simulink model "levitador_mpc_ss_delta"  (Simulink 7.9)
settings: Solver=ode5  SolverMode=SingleTasking  StartTime=0.0  StopTime=2  FixedStep=0.001  RelTol=1e-3
values from neighbouring files (symbols this model uses):
  C = [1 0]    [parametros_maglev_ss.m]
  g = 9.8    [parametros_maglev_ss.m]
  gamma = 328    [parametros_maglev_ss.m]
  i0 = 0.514    [parametros_maglev_ss.m]
  Kdelta = aux2(1,:)    [matrizes_ss_delta.m]
  Kf = 1.2e-4    (= 0.00012)    [parametros_maglev_ss.m]
  mass = 2.12e-2    (= 0.0212)    [parametros_maglev_ss.m]
  Nu = aux(end,:)    [matrizes_ss_delta.m]
  Nx = aux(1:n,:)    [matrizes_ss_delta.m]
  r = 0.166    [parametros_maglev_ss.m]
  T = 0.005    [parametros_maglev_ss.m]
  up_equilibrio = ( sqrt(mass*g/Kf)*(yp_equilibrio - y0) / gamma - i0 ) / r    [parametros_maglev_ss.m]
  y0 = -7.47    [parametros_maglev_ss.m]
  yp_equilibrio = 0    [parametros_maglev_ss.m]
undefined symbols (not defined in the file or in its folder): A, B
settings Model: Creator=Kawakami  LastModifiedBy=Kawakami
settings DataIOCC: SignalLoggingName=sigsOut
settings OptimizationCC: BooleanDataType=off
settings DebuggingCC: SaveWithParameterizedLinksMsg=none  SignalResolutionControl=TryResolveAllWithWarning  SolverPrmCheckMsg=none  MultiTaskDSMMsg=warning  MultiTaskCondExecSysMsg=none  FcnCallInpInsideContextMsg=Use local settings  StrictBusMsg=None
settings HardwareCC: TargetUnknown=on
settings RTWCC: IncludeERTFirstTime=on
settings GRTTargetCC: CombineOutputUpdateFcns=off  GRTInterface=on

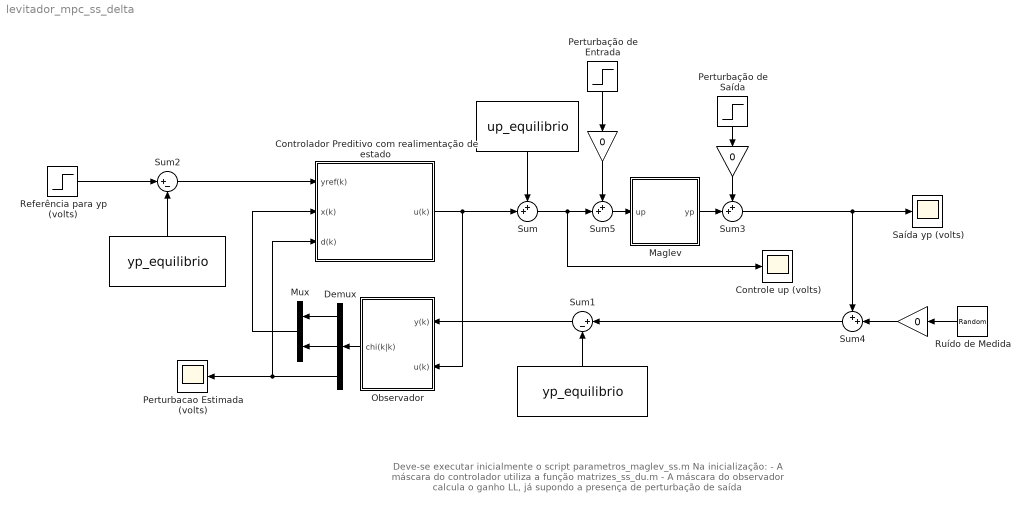
== system levitador_mpc_ss_delta ==
  note: Deve-se executar inicialmente o script parametros_maglev_ss.m
      |
      | Na inicialização:
      | - A máscara do controlador utiliza a função matrizes_ss_du.m
      | - A máscara do observador calcula o ganho LL, já supondo a presença de perturbação de saída
  " " : Constant  Value=yp_equilibrio
  "  " : Constant  Value=yp_equilibrio
  "   " : Constant  Value=up_equilibrio
  "     " : Gain  Gain=0
  "        " : Gain  Gain=0
  "         " : Gain  Gain=0
  Controlador Preditivo com realimentação de estado : Subsystem  mask{rho=1, N=20, M=5, A=A, B=B, C=C, T=T}
      mask prompts: rho "Peso do controle (rho)"; N "Horizonte de Predição (N)"; M "Horizonte de Controle (M)"; A "Matriz A"; B "Matriz B"; C "Matriz C"; T "Periodo de amostragem"
      mask init:
      | [Nx,Nu,Kdelta] = matrizes_ss_delta(A,B,C,N,M,rho);
  Controle up (volts) : Scope
      settings: TimeRange=2  YMin=2  YMax=3.5  SaveName=y1
  Demux : Demux  Outputs=3
  Maglev : Subsystem  mask{mass=mass, g=g, y0=y0, gamma=gamma, i0=i0, r=r, Kf=Kf, yp_inicial=yp_equilibrio, T=T}
      mask prompts: mass "massa (kg)"; g "g (m/s^2)"; y0 "y0 (V)"; gamma "gamma (V/m)"; i0 "i0 (A)"; r "r (A/V)"; Kf "Kf (N*m^2/A^2)"; yp_inicial "yp inicial (V)"; T "Periodo de Amostragem (s)"
  Mux : Mux  Inputs=2
  Observador : Subsystem  mask{A=A, B=B, C=C, T=T, poles=[0.5, 0.45, 0.4]}
      mask prompts: A "Matriz A"; B "Matriz B"; C "Matriz C"; T "Periodo de amostragem"; poles "Pólos para a dinâmica de erro de estimação"
      mask init:
      | n = size(A,1);
      | zerosn = zeros(n,1);
      | Ab = [A zerosn ; zerosn' 1];
      | Bb = [B;0];
      | Cb = [C 1];
      | L = place(Ab',Cb',poles)';
      | LL = inv(Ab)*L;
  Perturbacao Estimada (volts) : Scope
      settings: TimeRange=2  YMin=-0.4  YMax=1  SaveName=y2  SampleInput=on  SampleTime=T
  Perturbação de Entrada : Step  After=0.5  SampleTime=0
  Perturbação de Saída : Step  After=-0.1  SampleTime=0
  Referência para yp (volts) : Step  Time=0.2  After=0.5  SampleTime=0
  Ruído de Medida : RandomNumber  Variance=0.0001  SampleTime=0
  Saída yp (volts) : Scope
      settings: TimeRange=2  YMin=-0.1  YMax=0.9  SaveName=y
  Sum{,3..5} (4 alike) : Sum  Inputs=++|  SaturateOnIntegerOverflow=on
  Sum1 : Sum  Inputs=|+-  SaturateOnIntegerOverflow=on
  Sum2 : Sum  Inputs=|+-  SaturateOnIntegerOverflow=on
  wires:
  Controlador Preditivo com realimentação de estado/1(u(k)) -> Sum/2, Observador/2(u(k))
  Sum2/1 -> Controlador Preditivo com realimentação de estado/1(yref(k))
  Referência para yp (volts)/1 -> Sum2/1
  Maglev/1(yp) -> Sum3/2
  Sum3/1 -> Sum4/1, Saída yp (volts)/1
  Perturbação de Saída/1 -> "        "/1
  Sum/1 -> Sum5/2, Controle up (volts)/1
  Sum5/1 -> Maglev/1(up)
  Perturbação de Entrada/1 -> "     "/1
  Ruído de Medida/1 -> "         "/1
  Sum1/1 -> Observador/1(y(k))
  Observador/1(chi(k|k)) -> Demux/1
  Demux/3 -> Perturbacao Estimada (volts)/1, Controlador Preditivo com realimentação de estado/3(d(k))
  Sum4/1 -> Sum1/1
  "     "/1 -> Sum5/1
  "        "/1 -> Sum3/1
  "         "/1 -> Sum4/2
  "   "/1 -> Sum/1
  " "/1 -> Sum1/2
  "  "/1 -> Sum2/2
  Demux/1 -> Mux/1
  Demux/2 -> Mux/2
  Mux/1 -> Controlador Preditivo com realimentação de estado/2(x(k))

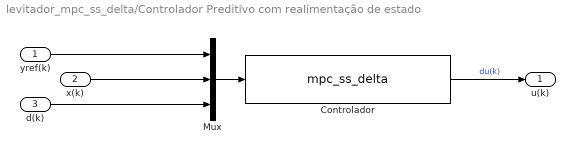
== system levitador_mpc_ss_delta/Controlador Preditivo com realimentação de estado ==
  yref(k) : Inport
  x(k) : Inport  Port=2
  d(k) : Inport  Port=3
  Controlador : S-Function  FunctionName=mpc_ss_delta  Parameters=Nx,Nu,Kdelta,T  EnableBusSupport=off
  Mux : Mux  Inputs=3
  u(k) : Outport
  wires:
  Mux/1 -> Controlador/1
  x(k)/1 -> Mux/2
  yref(k)/1 -> Mux/1
  Controlador/1 -> u(k)/1  "du(k)"
  d(k)/1 -> Mux/3

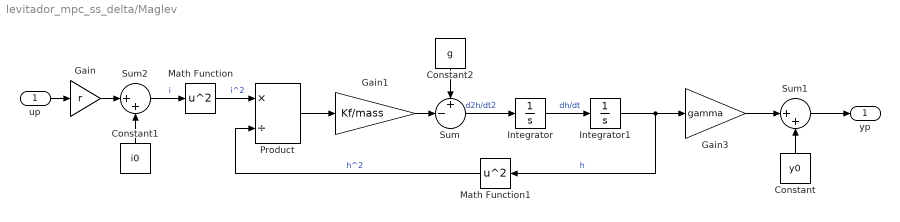
== system levitador_mpc_ss_delta/Maglev ==
  up : Inport
  Constant : Constant  Value=y0
  Constant1 : Constant  Value=i0
  Constant2 : Constant  Value=g
  Gain : Gain  Gain=r  SaturateOnIntegerOverflow=on  OutDataTypeStr=Inherit: Same as input  ParamDataTypeStr=Inherit: Same as input
  Gain1 : Gain  Gain=Kf/mass  SaturateOnIntegerOverflow=on  OutDataTypeStr=Inherit: Same as input  ParamDataTypeStr=Inherit: Same as input
  Gain3 : Gain  Gain=gamma  SaturateOnIntegerOverflow=on  OutDataTypeStr=Inherit: Same as input  ParamDataTypeStr=Inherit: Same as input
  Integrator : Integrator
  Integrator1 : Integrator  InitialCondition=(yp_inicial - y0)/gamma
  Math Function : Math  Operator=square  SaturateOnIntegerOverflow=on
  Math Function1 : Math  Operator=square  SaturateOnIntegerOverflow=on
  Product : Product  Inputs=*/  SaturateOnIntegerOverflow=on  OutDataTypeStr=Inherit: Same as first input
  Sum : Sum  Inputs=+-|  SaturateOnIntegerOverflow=on
  Sum1 : Sum  Inputs=|++  SaturateOnIntegerOverflow=on
  Sum2 : Sum  Inputs=|++  SaturateOnIntegerOverflow=on
  yp : Outport
  wires:
  Constant2/1 -> Sum/1
  Gain1/1 -> Sum/2
  Product/1 -> Gain1/1
  Math Function1/1 -> Product/2  "h^2"
  Math Function/1 -> Product/1  "i^2"
  Sum2/1 -> Math Function/1  "i"
  Gain/1 -> Sum2/1
  Constant1/1 -> Sum2/2
  Sum1/1 -> yp/1
  Gain3/1 -> Sum1/1
  Constant/1 -> Sum1/2
  up/1 -> Gain/1
  Integrator1/1 -> Math Function1/1, Gain3/1  "h"
  Sum/1 -> Integrator/1  "d2h/dt2"
  Integrator/1 -> Integrator1/1  "dh/dt"

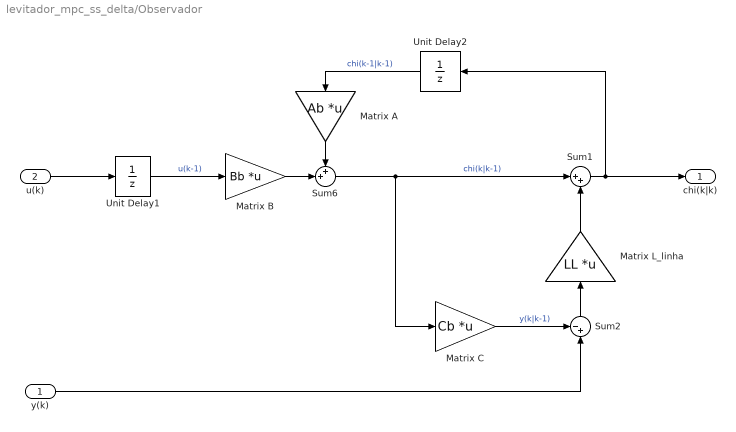
== system levitador_mpc_ss_delta/Observador ==
  y(k) : Inport
  u(k) : Inport  Port=2
  Matrix L_linha : Gain  Gain=LL  Multiplication=Matrix(K*u)  SaturateOnIntegerOverflow=on  OutDataTypeStr=Inherit: Same as input  ParamDataTypeStr=Inherit: Same as input
  Matrix A : Gain  Gain=Ab  Multiplication=Matrix(K*u)  SaturateOnIntegerOverflow=on  OutDataTypeStr=Inherit: Same as input  ParamDataTypeStr=Inherit: Same as input
  Matrix B : Gain  Gain=Bb  Multiplication=Matrix(K*u)  SaturateOnIntegerOverflow=on  OutDataTypeStr=Inherit: Same as input  ParamDataTypeStr=Inherit: Same as input
  Matrix C : Gain  Gain=Cb  Multiplication=Matrix(K*u)  SaturateOnIntegerOverflow=on  OutDataTypeStr=Inherit: Same as input  ParamDataTypeStr=Inherit: Same as input
  Sum1 : Sum  Inputs=|++  SaturateOnIntegerOverflow=on
  Sum2 : Sum  Inputs=-+|  SaturateOnIntegerOverflow=on
  Sum6 : Sum  Inputs=++|  SaturateOnIntegerOverflow=on
  Unit Delay1 : UnitDelay  SampleTime=T
  Unit Delay2 : UnitDelay  SampleTime=T
  chi(k|k) : Outport
  wires:
  u(k)/1 -> Unit Delay1/1
  Unit Delay1/1 -> Matrix B/1  "u(k-1)"
  Matrix B/1 -> Sum6/2
  Sum6/1 -> Sum1/1, Matrix C/1  "chi(k|k-1)"
  Sum1/1 -> Unit Delay2/1, chi(k|k)/1
  Matrix A/1 -> Sum6/1
  Unit Delay2/1 -> Matrix A/1  "chi(k-1|k-1)"
  Matrix L_linha/1 -> Sum1/2
  Sum2/1 -> Matrix L_linha/1
  Matrix C/1 -> Sum2/1  "y(k|k-1)"
  y(k)/1 -> Sum2/2
